simulink model "Sistema_completo_LTI_equiv"  (R2023b)
settings: Solver=VariableStepAuto  StartTime=0.0  StopTime=10.0  RelTol=1e-3
values from neighbouring files (symbols this model uses):
  b_eq = b_m + b_l/(r^2)    (= 2.19444444444e-05)    [polos_y_ceros.m]    (also in var1.m)
  C_ts = 0.818    [polos_y_ceros.m]    (also in var1.m)
  id0 = 1    [polos_y_ceros.m]    (also in var1.m)
  J_eq = J_m + J_l/(r^2)    (= 1.97847222222e-05)    [polos_y_ceros.m]    (also in var1.m = 4.58263888889e-05)
  L_d = 6.6 * 10^(-3)    (= 0.0066)    [polos_y_ceros.m]    (also in var1.m)
  L_q = 5.8 * 10^(-3)    (= 0.0058)    [polos_y_ceros.m]    (also in var1.m)
  lambda_m = 0.016    [polos_y_ceros.m]    (also in var1.m)
  P_p = 3    [polos_y_ceros.m]    (also in var1.m)
  r = 120/1    (= 120)    [polos_y_ceros.m]    (also in var1.m)
  R_sREF = 1.02    [polos_y_ceros.m]    (also in var1.m)
  R_ts_amb = 146.7    [polos_y_ceros.m]    (also in var1.m)
undefined symbols (not defined in the file or in its folder): magnitude
settings Model: Creator=tomas  LastModifiedBy=tomas

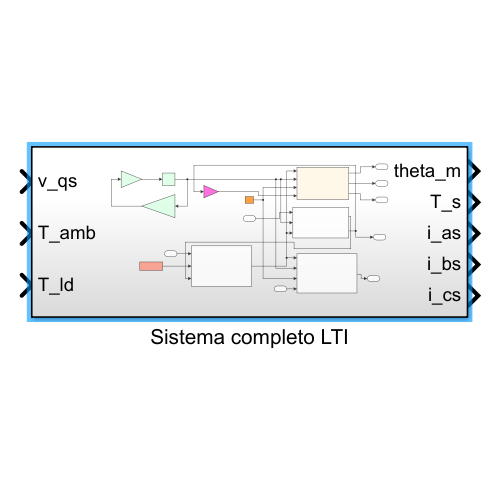
[thumbnail: Simulink's stored preview of the top-level diagram]
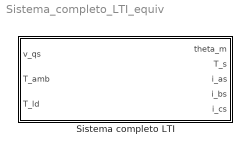
== system Sistema_completo_LTI_equiv ==
  Sistema completo LTI : Subsystem

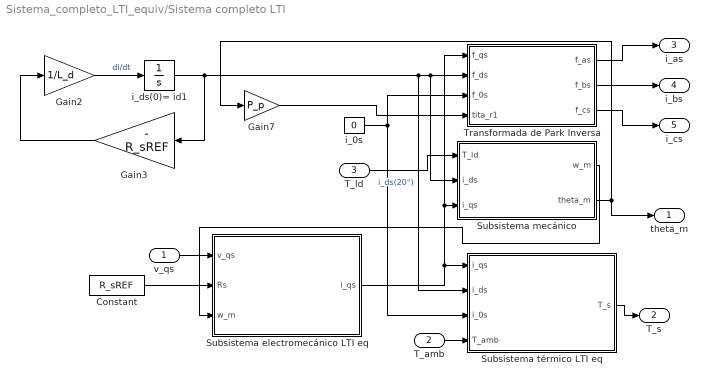
== system Sistema_completo_LTI_equiv/Sistema completo LTI ==
  v_qs : Inport
  T_amb : Inport  Port=2
  T_ld : Inport  Port=3
  Constant : Constant  Value=R_sREF
  Gain2 : Gain  Gain=1/L_d
  Gain3 : Gain  Gain=- R_sREF
  Gain7 : Gain  Gain=P_p
  Subsistema electromecánico LTI eq : Subsystem
  Subsistema mecánico : Subsystem
  Subsistema térmico LTI eq : Subsystem
  Transformada de Park Inversa : Subsystem
  i_0s : Constant  Value=0
  i_ds(0)= id1 : Integrator  InitialCondition=id0
  theta_m : Outport
  T_s : Outport  Port=2
  i_as : Outport  Port=3
  i_bs : Outport  Port=4
  i_cs : Outport  Port=5
  wires:
  Subsistema mecánico/2(theta_m) -> Gain7/1, theta_m/1
  v_qs/1 -> Subsistema electromecánico LTI eq/1(v_qs)
  Transformada de Park Inversa/1(f_as) -> i_as/1
  T_ld/1 -> Subsistema mecánico/1(T_ld)
  Transformada de Park Inversa/2(f_bs) -> i_bs/1
  Subsistema térmico LTI eq/1(T_s) -> T_s/1
  Transformada de Park Inversa/3(f_cs) -> i_cs/1
  Subsistema mecánico/1(w_m) -> Subsistema electromecánico LTI eq/3(w_m)
  T_amb/1 -> Subsistema térmico LTI eq/4(T_amb)
  i_0s/1 -> Subsistema térmico LTI eq/3(i_0s), Transformada de Park Inversa/3(f_0s)
  Constant/1 -> Subsistema electromecánico LTI eq/2(Rs)
  Subsistema electromecánico LTI eq/1(i_qs) -> Subsistema mecánico/3(i_qs), Transformada de Park Inversa/1(f_qs), Subsistema térmico LTI eq/1(i_qs)
  Gain7/1 -> Transformada de Park Inversa/4(tita_r1)
  i_ds(0)= id1/1 -> Transformada de Park Inversa/2(f_ds), Subsistema mecánico/2(i_ds), Subsistema térmico LTI eq/2(i_ds), Gain3/1  "i_ds(20°)"
  Gain2/1 -> i_ds(0)= id1/1  "di/dt"
  Gain3/1 -> Gain2/1

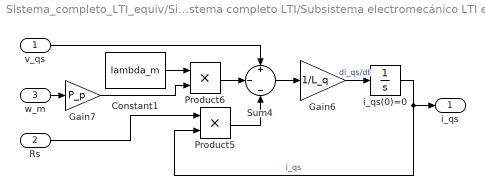
== system Sistema_completo_LTI_equiv/Sistema completo LTI/Subsistema electromecánico LTI eq ==
  v_qs : Inport
  Rs : Inport  Port=2
  w_m : Inport  Port=3
  Constant1 : Constant  Value=lambda_m
  Gain6 : Gain  Gain=1/L_q
  Gain7 : Gain  Gain=P_p
  Product5 : Product
  Product6 : Product
  Sum4 : Sum  Inputs=+|-|-
  i_qs(0)=0 : Integrator
  i_qs : Outport
  wires:
  i_qs(0)=0/1 -> i_qs/1, Product5/2  "i_qs"
  Constant1/1 -> Product6/1
  v_qs/1 -> Sum4/1
  Gain6/1 -> i_qs(0)=0/1  "di_qs/dt"
  Sum4/1 -> Gain6/1
  Rs/1 -> Product5/1
  w_m/1 -> Gain7/1
  Gain7/1 -> Product6/2
  Product5/1 -> Sum4/3
  Product6/1 -> Sum4/2

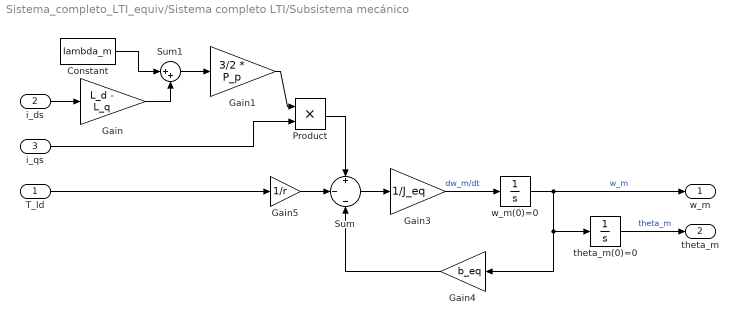
== system Sistema_completo_LTI_equiv/Sistema completo LTI/Subsistema mecánico ==
  T_ld : Inport
  i_ds : Inport  Port=2
  i_qs : Inport  Port=3
  Constant : Constant  Value=lambda_m
  Gain : Gain  Gain=L_d - L_q
  Gain1 : Gain  Gain=3/2 * P_p
  Gain3 : Gain  Gain=1/J_eq
  Gain4 : Gain  Gain=b_eq
  Gain5 : Gain  Gain=1/r
  Product : Product
  Sum : Sum  Inputs=+|-|-
  Sum1 : Sum  Inputs=|++
  theta_m(0)=0 : Integrator
  w_m(0)=0 : Integrator
  w_m : Outport
  theta_m : Outport  Port=2
  wires:
  w_m(0)=0/1 -> w_m/1, theta_m(0)=0/1, Gain4/1  "w_m"
  Sum/1 -> Gain3/1
  Gain3/1 -> w_m(0)=0/1  "dw_m/dt"
  T_ld/1 -> Gain5/1
  theta_m(0)=0/1 -> theta_m/1  "theta_m"
  i_ds/1 -> Gain/1
  Constant/1 -> Sum1/1
  Gain/1 -> Sum1/2
  Sum1/1 -> Gain1/1
  Gain1/1 -> Product/1
  i_qs/1 -> Product/2
  Product/1 -> Sum/1
  Gain4/1 -> Sum/3
  Gain5/1 -> Sum/2

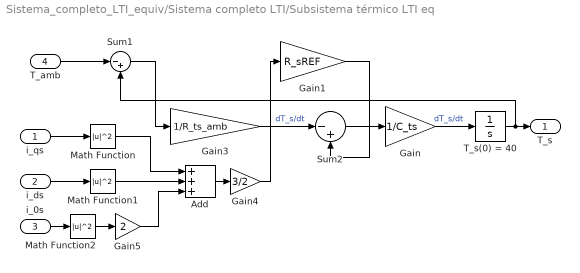
== system Sistema_completo_LTI_equiv/Sistema completo LTI/Subsistema térmico LTI eq ==
  i_qs : Inport
  i_ds : Inport  Port=2
  i_0s : Inport  Port=3
  T_amb : Inport  Port=4
  Add : Sum  Inputs=+++
  Gain : Gain  Gain=1/C_ts
  Gain1 : Gain  Gain=R_sREF
  Gain3 : Gain  Gain=1/R_ts_amb
  Gain4 : Gain  Gain=3/2
  Gain5 : Gain  Gain=2
  Math Function : Math  Operator=magnitude^2
  Math Function1 : Math  Operator=magnitude^2
  Math Function2 : Math  Operator=magnitude^2
  Sum1 : Sum  Inputs=|-+
  Sum2 : Sum  Inputs=|-+
  T_s(0) = 40 : Integrator  InitialCondition=40
  T_s : Outport
  wires:
  Math Function2/1 -> Gain5/1
  Math Function/1 -> Add/1
  T_amb/1 -> Sum1/1
  Sum2/1 -> Gain/1
  Sum1/1 -> Gain3/1
  Gain1/1 -> Sum2/2
  i_ds/1 -> Math Function1/1
  Gain/1 -> T_s(0) = 40/1  "dT_s/dt"
  Gain4/1 -> Gain1/1
  T_s(0) = 40/1 -> Sum1/2, T_s/1
  Math Function1/1 -> Add/2
  i_0s/1 -> Math Function2/1
  Add/1 -> Gain4/1
  Gain5/1 -> Add/3
  i_qs/1 -> Math Function/1
  Gain3/1 -> Sum2/1  "dT_s/dt"

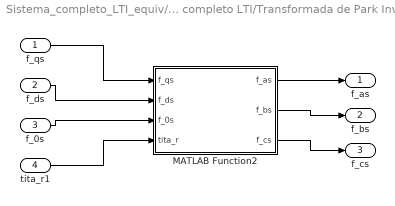
== system Sistema_completo_LTI_equiv/Sistema completo LTI/Transformada de Park Inversa ==
  f_qs : Inport
  f_ds : Inport  Port=2
  f_0s : Inport  Port=3
  tita_r1 : Inport  Port=4
  MATLAB Function2 : MATLAB Function  TreatAsAtomicUnit=on
  f_as : Outport
  f_bs : Outport  Port=2
  f_cs : Outport  Port=3
  wires:
  tita_r1/1 -> MATLAB Function2/4(tita_r)
  MATLAB Function2/2(f_bs) -> f_bs/1
  MATLAB Function2/1(f_as) -> f_as/1
  f_ds/1 -> MATLAB Function2/2(f_ds)
  MATLAB Function2/3(f_cs) -> f_cs/1
  f_0s/1 -> MATLAB Function2/3(f_0s)
  f_qs/1 -> MATLAB Function2/1(f_qs)

== matlab function Sistema_completo_LTI_equiv/Sistema completo LTI/Transformada de Park Inversa/MATLAB Function2 ==
  data: f_qs input; f_as output; f_ds input; f_0s input; tita_r input; f_bs output; f_cs output
function [f_as, f_bs, f_cs] = parkInv(f_qs,f_ds,f_0s,tita_r)

answer = [cos(tita_r), sin(tita_r), 1;
         cos(tita_r - 2*pi/3), sin(tita_r - 2*pi/3), 1;
         cos(tita_r + 2*pi/3), sin(tita_r + 2*pi/3), 1] * [f_qs;f_ds;f_0s]; 

f_as = answer(1);
f_bs = answer(2);
f_cs = answer(3);
